simulink model "Lecture1_Done_Simulink"  (R2022a)
settings: Solver=VariableStepAuto  StartTime=0.0  StopTime=45  RelTol=1e-3
libraries: simulink x1
settings Model: Creator=xuntang_lsu  LastModifiedBy=xuntang_lsu

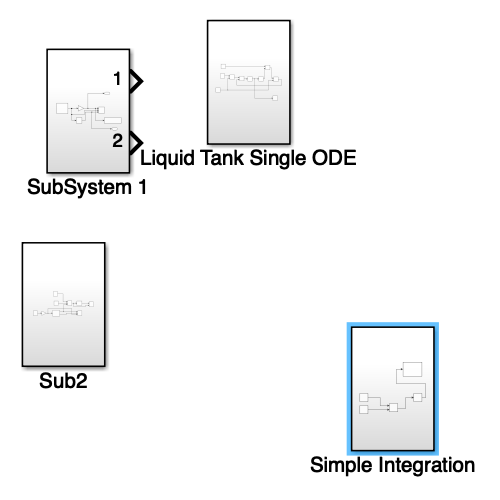
[thumbnail: Simulink's stored preview of the top-level diagram]
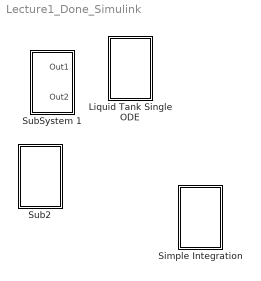
== system Lecture1_Done_Simulink ==
  Liquid Tank Single ODE : Subsystem
  Simple Integration : Subsystem
  Sub2 : Subsystem
  SubSystem 1 : Subsystem

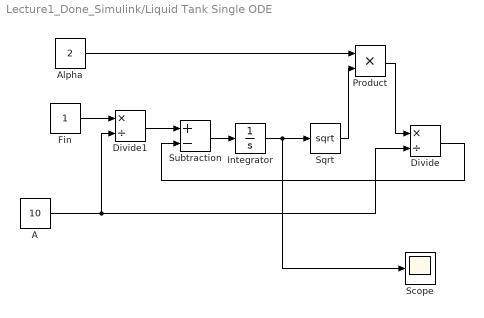
== system Lecture1_Done_Simulink/Liquid Tank Single ODE ==
  A : Constant  Value=10
  Alpha : Constant  Value=2
  Divide : Product  Inputs=*/
  Divide1 : Product  Inputs=*/
  Fin : Constant
  Integrator : Integrator  InitialCondition=0.5
  Product : Product
  Scope : Scope
  Sqrt : Sqrt
  Subtraction : Sum  Inputs=+-
  wires:
  Alpha/1 -> Product/1
  Fin/1 -> Divide1/1
  Divide1/1 -> Subtraction/1
  Subtraction/1 -> Integrator/1
  Sqrt/1 -> Product/2
  Divide/1 -> Subtraction/2
  Integrator/1 -> Sqrt/1, Scope/1
  A/1 -> Divide/2, Divide1/2
  Product/1 -> Divide/1

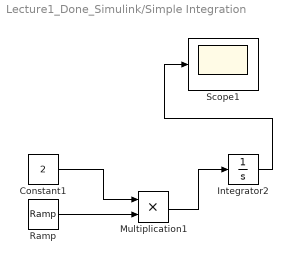
== system Lecture1_Done_Simulink/Simple Integration ==
  Constant1 : Constant  Value=2
  Integrator2 : Integrator
  Multiplication1 : Product  Inputs=**
  Ramp : simulink/Sources/Ramp  slope=1  start=0  InitialOutput=0
  Scope1 : Scope
  wires:
  Integrator2/1 -> Scope1/1
  Ramp/1 -> Multiplication1/2
  Multiplication1/1 -> Integrator2/1
  Constant1/1 -> Multiplication1/1

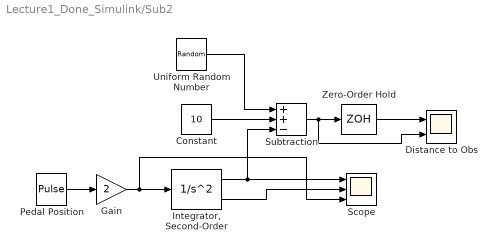
== system Lecture1_Done_Simulink/Sub2 ==
  Constant : Constant  Value=10
  Distance to Obs : Scope  NumInputPorts=2
  Gain : Gain  Gain=2
  "Integrator, Second-Order" : SecondOrderIntegrator  LimitX=on  UpperLimitX=5
  Pedal Position : DiscretePulseGenerator  PulseType=Time based  Period=10  PulseWidth=5
  Scope : Scope  NumInputPorts=3
  Subtraction : Sum  Inputs=++-
  Uniform Random Number : UniformRandomNumber  Minimum=-0.5  Maximum=0.5  SampleTime=0.1
  Zero-Order Hold : ZeroOrderHold
  wires:
  "Integrator, Second-Order"/1 -> Subtraction/3, Scope/1
  Zero-Order Hold/1 -> Distance to Obs/1
  Gain/1 -> Scope/3, "Integrator, Second-Order"/1
  Constant/1 -> Subtraction/2
  Uniform Random Number/1 -> Subtraction/1
  Pedal Position/1 -> Gain/1
  "Integrator, Second-Order"/2 -> Scope/2
  Subtraction/1 -> Distance to Obs/2, Zero-Order Hold/1

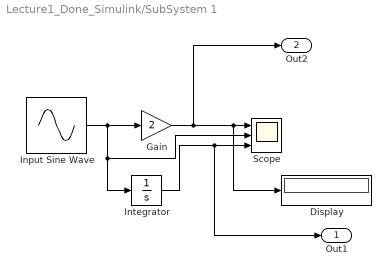
== system Lecture1_Done_Simulink/SubSystem 1 ==
  Display : Display
  Gain : Gain  Gain=2
  Input Sine Wave : Sin  SampleTime=0
  Integrator : Integrator
  Scope : Scope  NumInputPorts=3
  Out1 : Outport
  Out2 : Outport  Port=2
  wires:
  Integrator/1 -> Out1/1, Scope/3
  Input Sine Wave/1 -> Gain/1, Integrator/1, Scope/2
  Gain/1 -> Out2/1, Display/1, Scope/1
